simulink model "cartesian_pos"  (R2020a)
settings: Solver=VariableStepAuto  StartTime=0.0  StopTime=3  RelTol=1e-3
values from neighbouring files (symbols this model uses):
  Kp = wn^2*eye(2)    [cartesian_pos_control.m]
  Kv = 2*sqrt(Kp)*eye(2)    [cartesian_pos_control.m]
  Robot = SerialLink([links{:}], 'tool', transl([L(2), 0, 0]), 'name', 'Pacho Norras')    [robot.m]    (also in robotconfig.m)
  tstep = 0.02    [cartesian_pos_control.m]
  x0 = [1, -1]    [cartesian_pos_control.m]    (also in robotconfig.m = [1, -1, 0])
  xf = [1, 1]    [cartesian_pos_control.m]    (also in robotconfig.m = [1, 1, 0])
undefined symbols (not defined in the file or in its folder): coriolis
libraries: roblocks x14
settings Model: Creator=User  LastModifiedBy=cutig
settings SFSimCC: CustomCodeUndefinedFunction=UseInterfaceOnly

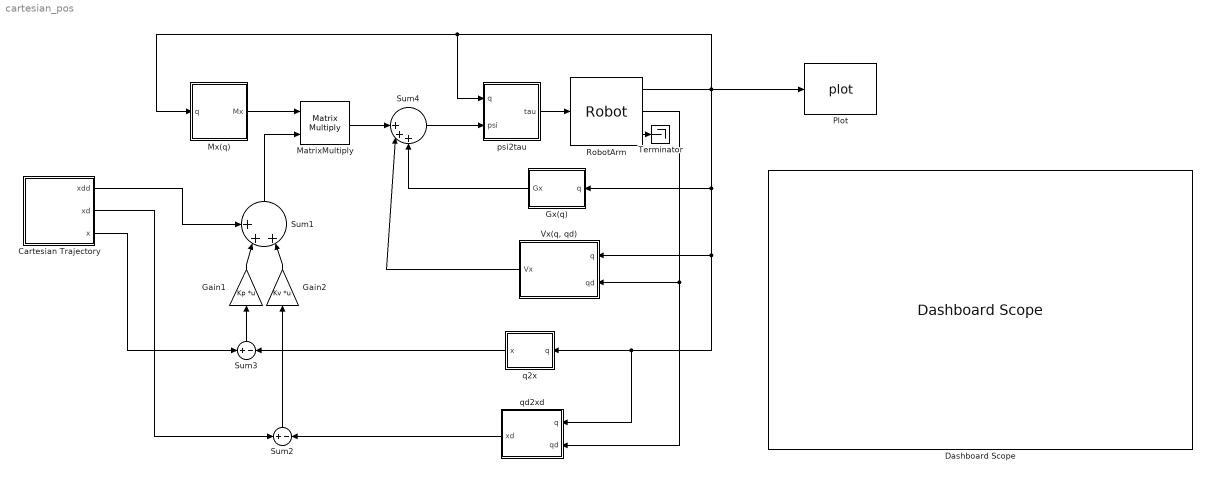
== system cartesian_pos ==
  Cartesian Trajectory : Subsystem  mask{initial_x=x0, final_x=xf, t_max=tf, ts=tstep}
      mask prompts: initial_x "Initial X"; final_x "Final X"; t_max "Maximum time"; ts "Timestep"
  Dashboard Scope : DashboardScope
  Gain1 : Gain  Gain=Kp  Multiplication=Matrix(K*u)
  Gain2 : Gain  Gain=Kv  Multiplication=Matrix(K*u)
  "Gx(q) " : Subsystem  mask{robot=Robot}
  MatrixMultiply : Product  Multiplication=Matrix(*)
  Mx(q) : Subsystem  mask{robot=Robot}
  Plot : roblocks/Arm/plot  robot=Robot  fps=30  holdplot=on
  RobotArm : roblocks/Arm/Robot  robot=Robot  q0=q0
  Sum1 : Sum  Inputs=+++|
  Sum2 : Sum  Inputs=+|-
  Sum3 : Sum  Inputs=+|-
  Sum4 : Sum  Inputs=||+++
  Terminator : Terminator
  "Vx(q, qd)" : Subsystem  mask{robot=Robot}
  psi2tau : Subsystem  mask{robot=Robot}
  q2x : Subsystem  mask{robot=Robot}
  qd2xd : Subsystem  mask{robot=Robot}
  wires:
  RobotArm/3 -> Terminator/1
  Sum4/1 -> psi2tau/2(psi)
  qd2xd/1(xd) -> Sum2/2
  Sum2/1 -> Gain2/1
  RobotArm/1 -> qd2xd/1(q), q2x/1(q), "Vx(q, qd)"/1(q), "Gx(q) "/1(q), Plot/1, Mx(q)/1(q), psi2tau/1(q)
  MatrixMultiply/1 -> Sum4/1
  RobotArm/2 -> qd2xd/2(qd), "Vx(q, qd)"/2(qd)
  Sum1/1 -> MatrixMultiply/2
  Gain1/1 -> Sum1/2
  Sum3/1 -> Gain1/1
  Gain2/1 -> Sum1/3
  Mx(q)/1(Mx) -> MatrixMultiply/1
  q2x/1(x) -> Sum3/2
  psi2tau/1(tau) -> RobotArm/1
  Cartesian Trajectory/1(xdd) -> Sum1/1
  Cartesian Trajectory/3(x) -> Sum3/1
  Cartesian Trajectory/2(xd) -> Sum2/1
  "Gx(q) "/1(Gx) -> Sum4/3
  "Vx(q, qd)"/1(Vx) -> Sum4/2

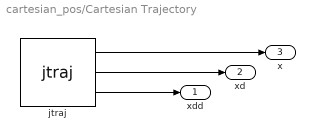
== system cartesian_pos/Cartesian Trajectory ==
  jtraj : roblocks/Toolbox/jtraj  q0=initial_x  qf=final_x  tmax=t_max  ts=ts
  xdd : Outport  VectorParamsAs1DForOutWhenUnconnected=off
  xd : Outport  Port=2  VectorParamsAs1DForOutWhenUnconnected=off
  x : Outport  Port=3  VectorParamsAs1DForOutWhenUnconnected=off
  wires:
  jtraj/2 -> xd/1
  jtraj/1 -> x/1
  jtraj/3 -> xdd/1

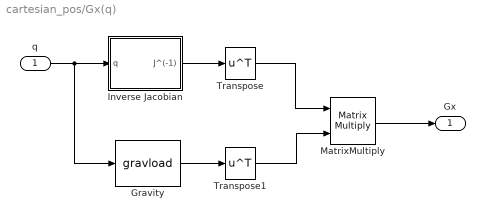
== system cartesian_pos/Gx(q)  ==
  q : Inport
  Gravity : roblocks/Arm/gravload  robot=Robot
  Inverse Jacobian : Subsystem  mask{robot=robot}
  MatrixMultiply : Product  Multiplication=Matrix(*)
  Transpose : Math  Operator=transpose  SignedPower=on  SaturateOnIntegerOverflow=on
  Transpose1 : Math  Operator=transpose  SignedPower=on  SaturateOnIntegerOverflow=on
  Gx : Outport  VectorParamsAs1DForOutWhenUnconnected=off
  wires:
  q/1 -> Gravity/1, Inverse Jacobian/1(q)
  Inverse Jacobian/1(J^(-1)) -> Transpose/1
  Transpose/1 -> MatrixMultiply/1
  Gravity/1 -> Transpose1/1
  MatrixMultiply/1 -> Gx/1
  Transpose1/1 -> MatrixMultiply/2

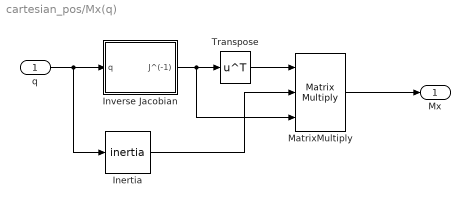
== system cartesian_pos/Mx(q) ==
  q : Inport
  Inertia : roblocks/Arm/inertia  robot=robot
  Inverse Jacobian : Subsystem  mask{robot=robot}
  MatrixMultiply : Product  Inputs=3  Multiplication=Matrix(*)
  Transpose : Math  Operator=transpose  SignedPower=on  SaturateOnIntegerOverflow=on
  Mx : Outport  VectorParamsAs1DForOutWhenUnconnected=off
  wires:
  MatrixMultiply/1 -> Mx/1
  q/1 -> Inertia/1, Inverse Jacobian/1(q)
  Inverse Jacobian/1(J^(-1)) -> MatrixMultiply/3, Transpose/1
  Transpose/1 -> MatrixMultiply/1
  Inertia/1 -> MatrixMultiply/2

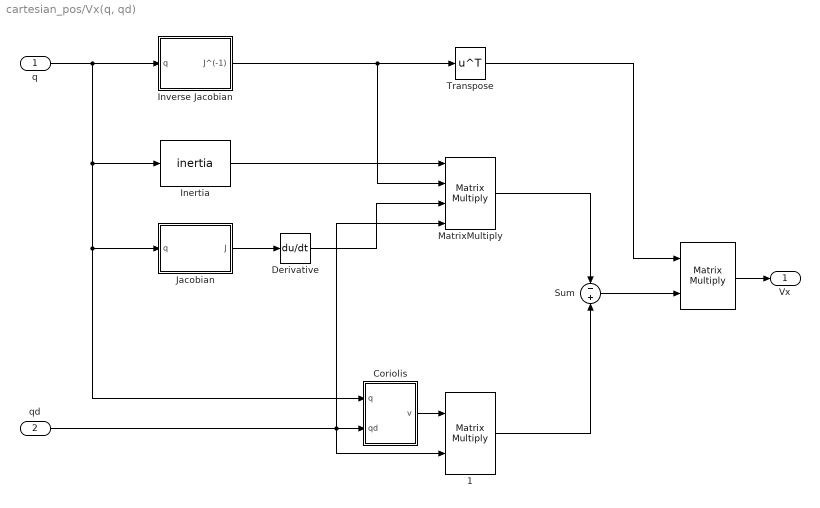
== system cartesian_pos/Vx(q, qd) ==
  q : Inport
  qd : Inport  Port=2
  " " : Product  Multiplication=Matrix(*)
  " 1" : Product  Multiplication=Matrix(*)
  Coriolis : Subsystem  mask{robot=robot}
  Derivative : Derivative
  Inertia : roblocks/Arm/inertia  robot=robot
  Inverse Jacobian : Subsystem  mask{robot=robot}
  Jacobian : Subsystem  mask{robot=robot}
  MatrixMultiply : Product  Inputs=4  Multiplication=Matrix(*)
  Sum : Sum  Inputs=-+
  Transpose : Math  Operator=transpose  SignedPower=on  SaturateOnIntegerOverflow=on
  Vx : Outport  VectorParamsAs1DForOutWhenUnconnected=off
  wires:
  " "/1 -> Vx/1
  qd/1 -> Coriolis/2(qd), MatrixMultiply/4, " 1"/2
  q/1 -> Inverse Jacobian/1(q), Coriolis/1(q), Jacobian/1(q), Inertia/1
  Inverse Jacobian/1(J^(-1)) -> MatrixMultiply/2, Transpose/1
  Transpose/1 -> " "/1
  Jacobian/1(J) -> Derivative/1
  Inertia/1 -> MatrixMultiply/1
  Derivative/1 -> MatrixMultiply/3
  Coriolis/1(v) -> " 1"/1
  MatrixMultiply/1 -> Sum/1
  Sum/1 -> " "/2
  " 1"/1 -> Sum/2

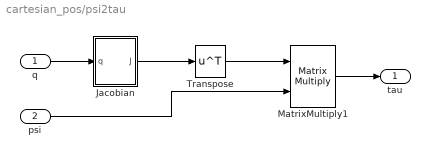
== system cartesian_pos/psi2tau ==
  q : Inport
  psi : Inport  Port=2
  Jacobian : Subsystem  mask{robot=robot}
  MatrixMultiply1 : Product  Multiplication=Matrix(*)
  Transpose : Math  Operator=transpose  SignedPower=on  SaturateOnIntegerOverflow=on
  tau : Outport  VectorParamsAs1DForOutWhenUnconnected=off
  wires:
  q/1 -> Jacobian/1(q)
  Jacobian/1(J) -> Transpose/1
  Transpose/1 -> MatrixMultiply1/1
  MatrixMultiply1/1 -> tau/1
  psi/1 -> MatrixMultiply1/2

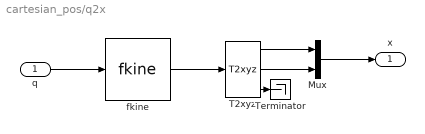
== system cartesian_pos/q2x ==
  q : Inport
  Mux : Mux  Inputs=2
  T2xyz : roblocks/Toolbox/T2xyz
  Terminator : Terminator
  fkine : roblocks/Arm/fkine  robot=robot
  x : Outport  VectorParamsAs1DForOutWhenUnconnected=off
  wires:
  q/1 -> fkine/1
  fkine/1 -> T2xyz/1
  Mux/1 -> x/1
  T2xyz/1 -> Mux/1
  T2xyz/2 -> Mux/2
  T2xyz/3 -> Terminator/1

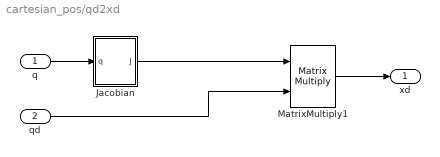
== system cartesian_pos/qd2xd ==
  q : Inport
  qd : Inport  Port=2
  Jacobian : Subsystem  mask{robot=robot}
  MatrixMultiply1 : Product  Multiplication=Matrix(*)
  xd : Outport  VectorParamsAs1DForOutWhenUnconnected=off
  wires:
  q/1 -> Jacobian/1(q)
  Jacobian/1(J) -> MatrixMultiply1/1
  MatrixMultiply1/1 -> xd/1
  qd/1 -> MatrixMultiply1/2

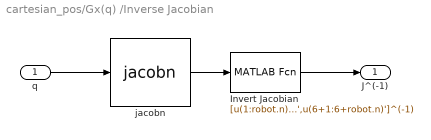
== system cartesian_pos/Gx(q) /Inverse Jacobian ==
  q : Inport
  Invert Jacobian : MATLABFcn  MATLABFcn=[u(1:robot.n)',u(6+1:6+robot.n)']^(-1)  OutputDimensions=[robot.n, robot.n]  Output1D=off
  jacobn : roblocks/Arm/jacobn  robot=robot
  J^(-1) : Outport  VectorParamsAs1DForOutWhenUnconnected=off
  wires:
  jacobn/1 -> Invert Jacobian/1
  q/1 -> jacobn/1
  Invert Jacobian/1 -> J^(-1)/1

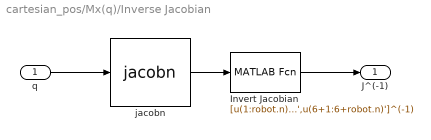
== system cartesian_pos/Mx(q)/Inverse Jacobian ==
  q : Inport
  Invert Jacobian : MATLABFcn  MATLABFcn=[u(1:robot.n)',u(6+1:6+robot.n)']^(-1)  OutputDimensions=[robot.n, robot.n]  Output1D=off
  jacobn : roblocks/Arm/jacobn  robot=robot
  J^(-1) : Outport  VectorParamsAs1DForOutWhenUnconnected=off
  wires:
  Invert Jacobian/1 -> J^(-1)/1
  q/1 -> jacobn/1
  jacobn/1 -> Invert Jacobian/1

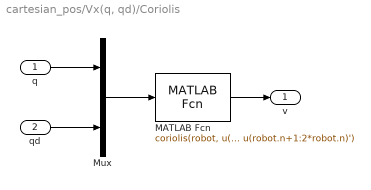
== system cartesian_pos/Vx(q, qd)/Coriolis ==
  q : Inport
  qd : Inport  Port=2
  MATLAB Fcn : MATLABFcn  MATLABFcn=coriolis(robot, u(1:robot.n)', u(robot.n+1:2*robot.n)')  OutputDimensions=[robot.n, robot.n]  Output1D=off
  Mux : Mux  Inputs=2
  v : Outport  VectorParamsAs1DForOutWhenUnconnected=off
  wires:
  qd/1 -> Mux/2
  MATLAB Fcn/1 -> v/1
  Mux/1 -> MATLAB Fcn/1
  q/1 -> Mux/1

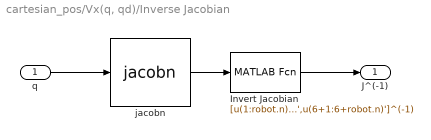
== system cartesian_pos/Vx(q, qd)/Inverse Jacobian ==
  q : Inport
  Invert Jacobian : MATLABFcn  MATLABFcn=[u(1:robot.n)',u(6+1:6+robot.n)']^(-1)  OutputDimensions=[robot.n, robot.n]  Output1D=off
  jacobn : roblocks/Arm/jacobn  robot=robot
  J^(-1) : Outport  VectorParamsAs1DForOutWhenUnconnected=off
  wires:
  jacobn/1 -> Invert Jacobian/1
  q/1 -> jacobn/1
  Invert Jacobian/1 -> J^(-1)/1

== system cartesian_pos/Vx(q, qd)/Jacobian ==
  q : Inport
  Slice : MATLABFcn  MATLABFcn=[u(1:robot.n)',u(6+1:6+robot.n)']  OutputDimensions=[robot.n, robot.n]  Output1D=off
  jacobn : roblocks/Arm/jacobn  robot=robot
  J : Outport  VectorParamsAs1DForOutWhenUnconnected=off
  wires:
  q/1 -> jacobn/1
  jacobn/1 -> Slice/1
  Slice/1 -> J/1

== system cartesian_pos/psi2tau/Jacobian ==
  q : Inport
  Slice : MATLABFcn  MATLABFcn=[u(1:robot.n)',u(6+1:6+robot.n)']  OutputDimensions=[robot.n, robot.n]  Output1D=off
  jacobn : roblocks/Arm/jacobn  robot=robot
  J : Outport  VectorParamsAs1DForOutWhenUnconnected=off
  wires:
  q/1 -> jacobn/1
  jacobn/1 -> Slice/1
  Slice/1 -> J/1

== system cartesian_pos/qd2xd/Jacobian ==
  q : Inport
  Slice : MATLABFcn  MATLABFcn=[u(1:robot.n)',u(6+1:6+robot.n)']  OutputDimensions=[robot.n, robot.n]  Output1D=off
  jacobn : roblocks/Arm/jacobn  robot=robot
  J : Outport  VectorParamsAs1DForOutWhenUnconnected=off
  wires:
  q/1 -> jacobn/1
  jacobn/1 -> Slice/1
  Slice/1 -> J/1
